simulink library "auroraNDILibrary"  (R2023a)
settings: Solver=VariableStepAuto  StartTime=0.0  StopTime=10.0  RelTol=1e-3
settings Model: Creator=Chris  LastModifiedBy=86188
settings DebuggingCC: UnconnectedInputMsg=warning  UnconnectedOutputMsg=warning  UnconnectedLineMsg=warning
settings ModelReferenceCC: EnableRefExpFcnMdlSchedulingChecks=on
settings RTWCC: DLArmComputeVersion=19.05

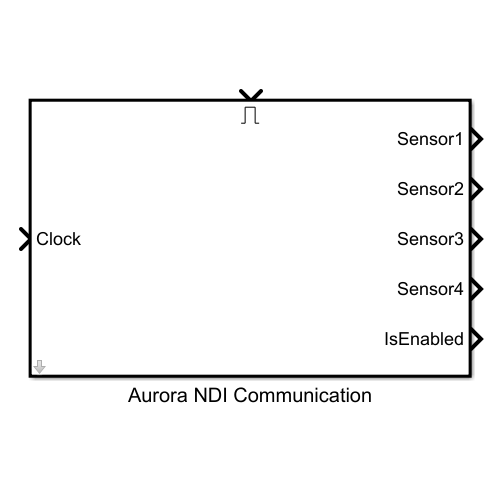
[thumbnail: Simulink's stored preview of the top-level diagram]
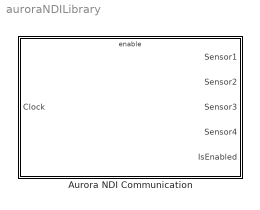
== system auroraNDILibrary ==
  Aurora NDI Communication : Subsystem  mask(Aurora NDI Communication){SampleFrequency=20, comNumber=0}
      mask prompts: SampleFrequency "Sample Frequency (Hz)"; comNumber "Port Number (Ex. "Com6", enter "6")"
      mask help: This block communicates with the Aurora NDI EM tracker. Sample frequency can be up to 40Hz as that is the hardware limit of the device. When running in Normal or Accelerator mode it has been found that the block can run up to ~20 Hz before the model can no longer keep pace.

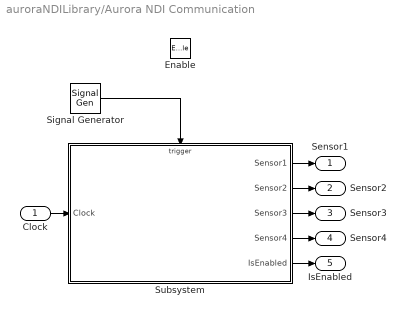
== system auroraNDILibrary/Aurora NDI Communication ==
  Clock : Inport
  Enable : EnablePort
  Signal Generator : SignalGenerator  WaveForm=square  Frequency=SampleFrequency
  Subsystem : Subsystem
  Sensor1 : Outport
  Sensor2 : Outport  Port=2
  Sensor3 : Outport  Port=3
  Sensor4 : Outport  Port=4
  IsEnabled : Outport  Port=5
  wires:
  Clock/1 -> Subsystem/1(Clock)
  Subsystem/3(Sensor3) -> Sensor3/1
  Subsystem/2(Sensor2) -> Sensor2/1
  Subsystem/1(Sensor1) -> Sensor1/1
  Subsystem/4(Sensor4) -> Sensor4/1
  Subsystem/5(IsEnabled) -> IsEnabled/1
  Signal Generator/1 -> Subsystem/Trigger

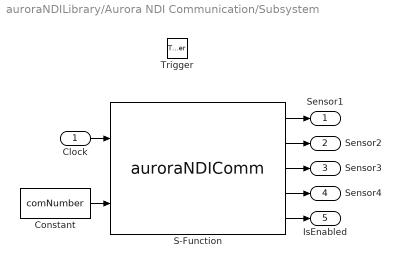
== system auroraNDILibrary/Aurora NDI Communication/Subsystem ==
  Clock : Inport
  Trigger : TriggerPort  VariantControl=(inherit)  PortDimensions=1
  Constant : Constant  Value=comNumber
  S-Function : S-Function  FunctionName=auroraNDIComm  SFunctionDeploymentMode=off  EnableBusSupport=off
  Sensor1 : Outport
  Sensor2 : Outport  Port=2
  Sensor3 : Outport  Port=3
  Sensor4 : Outport  Port=4
  IsEnabled : Outport  Port=5
  wires:
  S-Function/5 -> IsEnabled/1
  Clock/1 -> S-Function/1
  S-Function/3 -> Sensor3/1
  S-Function/4 -> Sensor4/1
  S-Function/2 -> Sensor2/1
  S-Function/1 -> Sensor1/1
  Constant/1 -> S-Function/2
